simulink model "controller_sim"  (R2012a)
settings: Solver=ode45  SolverMode=SingleTasking  StartTime=0.0  StopTime=5  MaxStep=.01  RelTol=1e-3
values from neighbouring files (symbols this model uses):
  bang_bang = true    [controller.m]
  external_bias = false    [controller.m]
  F_k = i_nl / k    (= 0.5)    [controller.m]
  I = .1    (= 0.1)    [controller.m]
  k = i_stall / t_stall    (= 0.4)    [controller.m]
  Kd = 0    [controller.m]
  Ki = 0    [controller.m]
  Kp = 1    [controller.m]
  R = V / i_stall    (= 2.14285714286)    [controller.m]
  step_input = true    [controller.m]
  supply_voltage = 1    [controller.m]
libraries: simulink x1
settings Model: CovMetricSettings=dwe  CovHtmlReporting=off  covSaveCumulativeToWorkspaceVar=off  CovSaveSingleToWorkspaceVar=off  CovExternalEMLEnable=on  Creator=Josh  LastModifiedBy=Brian
settings SolverCC: ZeroCrossControl=DisableAll  ZeroCrossAlgorithm=Adaptive
settings DataIOCC: SaveFormat=StructureWithTime
settings OptimizationCC: LifeSpan=inf  SimCompilerOptimization=Off
settings DebuggingCC: FcnCallInpInsideContextMsg=Enable All
settings HardwareCC: ProdWordSize=32  ProdHWDeviceType=Specified
settings RTWCC: RTWCompilerOptimization=Off
settings GRTTargetCC: CodeReplacementLibrary=C99 (ISO)  CPPClassGenCompliant=off

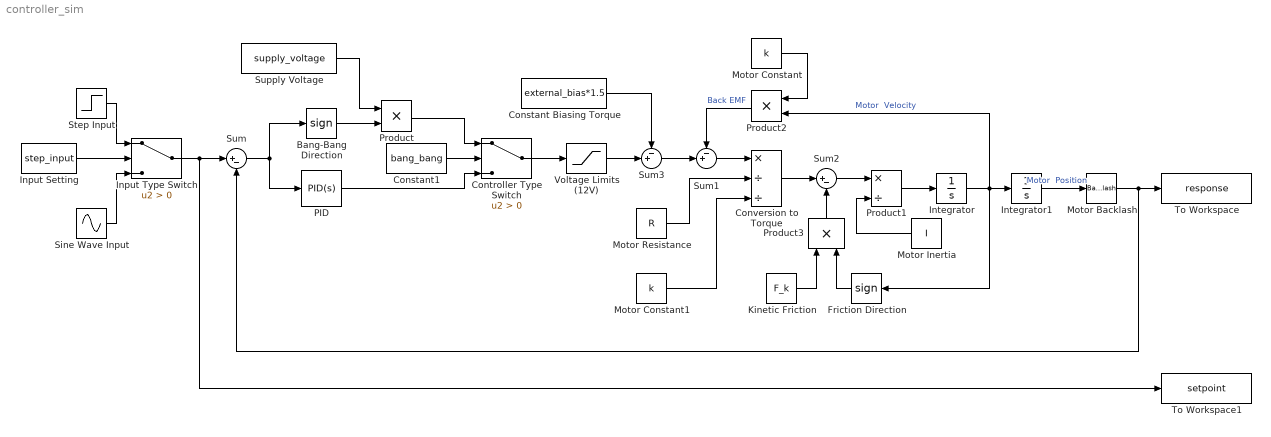
== system controller_sim ==
  " Motor Backlash" : Backlash  BacklashWidth=.01
  Bang-Bang Direction : Signum
  Constant Biasing Torque : Constant  Value=external_bias*1.5
  Constant1 : Constant  Value=bang_bang
  Controller Type Switch : Switch  Criteria=u2 > Threshold  ZeroCross=off
  Conversion to Torque : Product  Inputs=*//
  Friction Direction : Signum  ZeroCross=off
  Input Type Switch : Switch  Criteria=u2 > Threshold
  Input Setting : Constant  Value=step_input
  Integrator : Integrator
  Integrator1 : Integrator
  Kinetic Friction : Constant  Value=F_k
  Motor Inertia : Constant  Value=I
  Motor Resistance : Constant  Value=R
  Motor Constant1 : Constant  Value=k
  Motor Constant : Constant  Value=k
  "PID " : simulink/Continuous/PID Controller  Controller=PID  Form=Parallel  TimeDomain=Continuous-time  SampleTime=-1  IntegratorMethod=Forward Euler  FilterMethod=Forward Euler  ControllerParametersSource=internal  P=Kp  I=Ki  D=Kd  UseFilter=on  N=100  InitialConditionSource=internal  InitialConditionForIntegrator=0  InitialConditionForFilter=0  DifferentiatorICPrevScaledInput=0  ExternalReset=none  TrackingMode=off  Kt=1  LimitOutput=off  UpperSaturationLimit=inf  LowerSaturationLimit=-inf  LinearizeAsGain=on  AntiWindupMode=none  Kb=1  POutMin=[]  POutMax=[]  IOutMin=[]  IOutMax=[]  DOutMin=[]  DOutMax=[]  NOutMin=[]  NOutMax=[]  SumOutMin=[]  SumOutMax=[]  SaturationOutMin=[]  SaturationOutMax=[]  PParamMin=[]  PParamMax=[]  IParamMin=[]  IParamMax=[]  DParamMin=[]  DParamMax=[]  NParamMin=[]  NParamMax=[]  KbParamMin=[]  KbParamMax=[]  KtParamMin=[]  KtParamMax=[]  KbOutMin=[]  KbOutMax=[]  KtOutMin=[]  KtOutMax=[]  IntegratorOutMin=[]  IntegratorOutMax=[]  FilterOutMin=[]  FilterOutMax=[]  SumI1OutMin=[]  SumI1OutMax=[]  SumI2OutMin=[]  SumI2OutMax=[]  SumI3OutMin=[]  SumI3OutMax=[]  SumDOutMin=[]  SumDOutMax=[]  DifferentiatorOutMin=[]  DifferentiatorOutMax=[]  IntegratorContinuousStateAttributes=''  IntegratorStateMustResolveToSignalObject=off  IntegratorRTWStateStorageClass=Auto  FilterContinuousStateAttributes=''  FilterStateMustResolveToSignalObject=off  FilterRTWStateStorageClass=Auto
  Product : Product
  Product1 : Product  Inputs=*/
  Product2 : Product
  Product3 : Product  Inputs=**
  Sine Wave Input : Sin  Frequency=2*pi / 2.5  SampleTime=0
  Step Input : Step  Time=0  SampleTime=0
  Sum : Sum  Inputs=|+-
  Sum1 : Sum  Inputs=-+|
  Sum2 : Sum  Inputs=|+-
  Sum3 : Sum  Inputs=-+|
  Supply Voltage : Constant  Value=supply_voltage
  To Workspace : ToWorkspace  VariableName=response  SaveFormat=Timeseries  SampleTime=-1
  To Workspace1 : ToWorkspace  VariableName=setpoint  SaveFormat=Timeseries  SampleTime=-1
  Voltage Limits (12V) : Saturate  UpperLimit=12  LowerLimit=-12  ZeroCross=off
  wires:
  " Motor Backlash"/1 -> Sum/2, To Workspace/1
  Sum/1 -> Bang-Bang Direction/1, "PID "/1
  Bang-Bang Direction/1 -> Product/2
  Supply Voltage/1 -> Product/1
  "PID "/1 -> Controller Type Switch/3
  Controller Type Switch/1 -> Voltage Limits (12V)/1
  Product/1 -> Controller Type Switch/1
  Input Type Switch/1 -> To Workspace1/1, Sum/1
  Constant1/1 -> Controller Type Switch/2
  Sine Wave Input/1 -> Input Type Switch/3
  Input Setting/1 -> Input Type Switch/2
  Step Input/1 -> Input Type Switch/1
  Sum1/1 -> Conversion to Torque/1
  Integrator/1 -> Product2/2, Integrator1/1, Friction Direction/1  "Motor  Velocity"
  Product2/1 -> Sum1/1  "Back EMF"
  Motor Constant/1 -> Product2/1
  Motor Constant1/1 -> Conversion to Torque/3
  Motor Resistance/1 -> Conversion to Torque/2
  Product1/1 -> Integrator/1
  Motor Inertia/1 -> Product1/2
  Kinetic Friction/1 -> Product3/1
  Sum2/1 -> Product1/1
  Integrator1/1 -> " Motor Backlash"/1  "Motor  Position"
  Friction Direction/1 -> Product3/2
  Product3/1 -> Sum2/2
  Conversion to Torque/1 -> Sum2/1
  Voltage Limits (12V)/1 -> Sum3/2
  Sum3/1 -> Sum1/2
  Constant Biasing Torque/1 -> Sum3/1
